simulink library "component_lib"  (R2023a)
settings: Solver=VariableStepAuto  StartTime=0.0  StopTime=10.0  RelTol=1e-3
undefined symbols (not defined in the file or in its folder): ECCV_r, par, R1234yf_ph, V_nom
libraries: base_lib x258, $bdroot x212, simulink x2, slpidlib x1
(part 6 of 7)

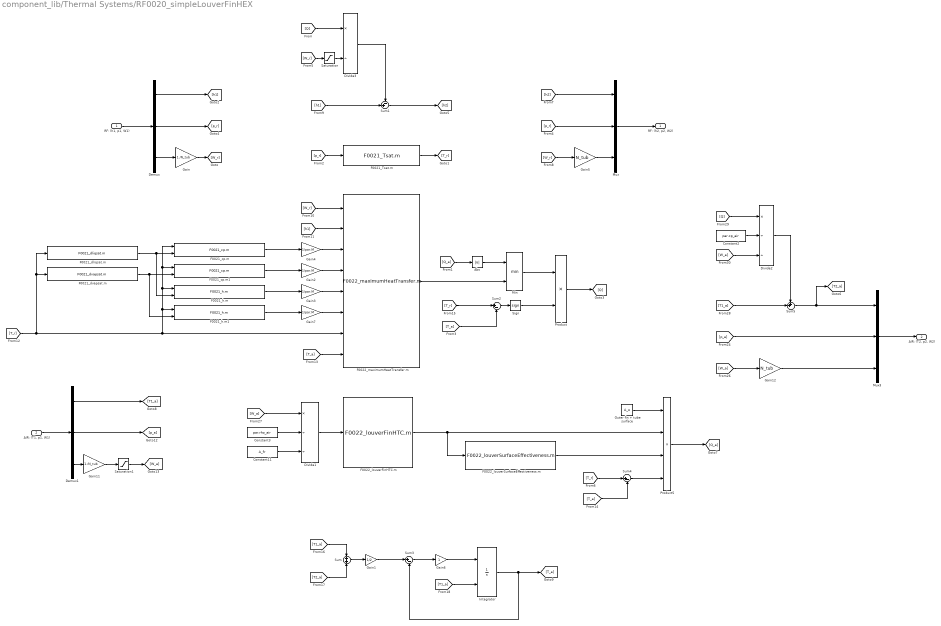
== system component_lib/Thermal Systems/RF0020_simpleLouverFinHEX ==
  "RF: (h1, p1, W1)" : Inport
  "AIR: (T1, p1, W1)" : Inport  Port=2
  Abs : Abs  SaturateOnIntegerOverflow=off
  Constant11 : Constant  Value=A_fr
  Constant2 : Constant  Value=par.cp_air
  Constant3 : Constant  Value=par.rho_air
  Demux : Demux  Outputs=3
  Demux1 : Demux  Outputs=3
  Divide1 : Product  Inputs=*//
  Divide2 : Product  Inputs=*//
  Divide3 : Product  Inputs=*/
  F0021_Tsat.m : base_lib/F0021_R1234yf/F0021_Tsat.m  SystemSampleTime=-1  VariantActivationTime=update diagram  Latency=0  AutoFrameSizeCalculation=off
      settings: LibrarySourceBlock=|
      | simulink/User-Defined
      | Functions/MATLAB Function
  F0021_cp.m : base_lib/F0021_R1234yf/F0021_cp.m  SystemSampleTime=-1  VariantActivationTime=update diagram  Latency=0  AutoFrameSizeCalculation=off
      settings: LibrarySourceBlock=|
      | simulink/User-Defined
      | Functions/MATLAB Function
  F0021_cp.m1 : base_lib/F0021_R1234yf/F0021_cp.m  SystemSampleTime=-1  VariantActivationTime=update diagram  Latency=0  AutoFrameSizeCalculation=off
      settings: LibrarySourceBlock=|
      | simulink/User-Defined
      | Functions/MATLAB Function
  F0021_dliqsat.m : base_lib/F0021_R1234yf/F0021_dliqsat.m  SystemSampleTime=-1  VariantActivationTime=update diagram  Latency=0  AutoFrameSizeCalculation=off
      settings: LibrarySourceBlock=|
      | simulink/User-Defined
      | Functions/MATLAB Function
  F0021_dvapsat.m : base_lib/F0021_R1234yf/F0021_dvapsat.m  SystemSampleTime=-1  VariantActivationTime=update diagram  Latency=0  AutoFrameSizeCalculation=off
      settings: LibrarySourceBlock=|
      | simulink/User-Defined
      | Functions/MATLAB Function
  F0021_h.m : base_lib/F0021_R1234yf/F0021_h.m  SystemSampleTime=-1  VariantActivationTime=update diagram  Latency=0  AutoFrameSizeCalculation=off
      settings: LibrarySourceBlock=|
      | simulink/User-Defined
      | Functions/MATLAB Function
  F0021_h.m1 : base_lib/F0021_R1234yf/F0021_h.m  SystemSampleTime=-1  VariantActivationTime=update diagram  Latency=0  AutoFrameSizeCalculation=off
      settings: LibrarySourceBlock=|
      | simulink/User-Defined
      | Functions/MATLAB Function
  F0022_louverFinHTC.m : base_lib/F0022_heatPump/F0022_louverFinHTC.m  SystemSampleTime=-1  VariantActivationTime=update diagram  Latency=0  AutoFrameSizeCalculation=off
      settings: LibrarySourceBlock=|
      | simulink/User-Defined
      | Functions/MATLAB Function
  F0022_louverSurfaceEffectiveness.m : base_lib/F0022_heatPump/F0022_louverSurfaceEffectiveness.m  SystemSampleTime=-1  VariantActivationTime=update diagram  Latency=0  AutoFrameSizeCalculation=off
      settings: LibrarySourceBlock=|
      | simulink/User-Defined
      | Functions/MATLAB Function
  F0022_maximumHeatTransfer.m : base_lib/F0022_heatPump/F0022_maximumHeatTransfer.m  SystemSampleTime=-1  VariantActivationTime=update diagram  Latency=0  AutoFrameSizeCalculation=off
      settings: LibrarySourceBlock=|
      | simulink/User-Defined
      | Functions/MATLAB Function
  Gain : Gain  Gain=1./N_tub
  Gain1 : Gain  Gain=1/2
  Gain11 : Gain  Gain=1./N_tub
  Gain12 : Gain  Gain=N_tub
  Gain{2..4,7} (4 alike) : Gain  Gain=1/par.M
  Gain5 : Gain  Gain=N_tub
  Gain6 : Gain
  Integrator : Integrator  InitialConditionSource=external  LimitOutput=on  UpperSaturationLimit=273+100  LowerSaturationLimit=273-40
  Min : MinMax  Inputs=2
  Mux : Mux  Inputs=3
  Mux3 : Mux  Inputs=3
  Outer fin + tube surface : Constant  Value=A_o
  Product : Product
  Product5 : Product  Inputs=4
  Saturation : Saturate  UpperLimit=inf  LowerLimit=1e-5
  Saturation1 : Saturate  UpperLimit=inf  LowerLimit=1e-3
  Sign : Signum
  Sum : Sum  Inputs=+|+
  Sum1 : Sum  Inputs=-+|
  Sum2 : Sum  Inputs=|+-
  Sum3 : Sum  Inputs=|+-
  Sum4 : Sum  Inputs=|+-
  Sum5 : Sum  Inputs=++|
  "RF: (h2, p2, W2)" : Outport
  "AIR: (T2, p2, W2)" : Outport  Port=2
  wires:
  [h2] -> Mux/1
  Gain5/1 -> Mux/3
  Demux/1 -> [h1]
  Demux/3 -> Gain/1
  Mux3/1 -> "AIR: (T2, p2, W2)"/1
  "AIR: (T1, p1, W1)"/1 -> Demux1/1
  Gain/1 -> [W_r]
  [p_r] -> Mux/2
  Demux/2 -> [p_r]
  [W_r] -> Gain5/1
  Mux/1 -> "RF: (h2, p2, W2)"/1
  "RF: (h1, p1, W1)"/1 -> Demux/1
  F0022_louverFinHTC.m/1 -> Product5/2, F0022_louverSurfaceEffectiveness.m/1
  Divide1/1 -> F0022_louverFinHTC.m/1
  Constant3/1 -> Divide1/2
  Constant11/1 -> Divide1/3
  Product5/1 -> [Q_a]
  Outer fin + tube surface/1 -> Product5/1
  [T_a] -> Sum4/2
  Sum4/1 -> Product5/4
  F0022_louverSurfaceEffectiveness.m/1 -> Product5/3
  Demux1/1 -> [T1_a]
  Demux1/2 -> [p_a]
  [p_a] -> Mux3/2
  Demux1/3 -> Gain11/1
  [W_a] -> Divide1/1
  Gain12/1 -> Mux3/3
  Gain11/1 -> Saturation1/1
  [W_a] -> Gain12/1
  [T1_a] -> Sum5/2
  Sum5/1 -> [T2_a], Mux3/1
  [Q] -> Divide2/1
  Constant2/1 -> Divide2/2
  [W_a] -> Divide2/3
  Divide2/1 -> Sum5/1
  Saturation1/1 -> [W_a]
  [p_r] -> F0021_Tsat.m/1
  F0021_Tsat.m/1 -> [T_r]
  [T_r] -> Sum4/1
  [Q] -> Divide3/1
  [h1] -> Sum1/2
  Divide3/1 -> Sum1/1
  Sum1/1 -> [h2]
  [W_r] -> F0022_maximumHeatTransfer.m/1
  [h1] -> F0022_maximumHeatTransfer.m/2
  Gain4/1 -> F0022_maximumHeatTransfer.m/3
  Gain2/1 -> F0022_maximumHeatTransfer.m/4
  F0021_cp.m/1 -> Gain4/1
  F0021_cp.m1/1 -> Gain2/1
  F0021_dliqsat.m/1 -> F0021_h.m/2, F0021_cp.m/2
  F0021_dvapsat.m/1 -> F0021_h.m1/2, F0021_cp.m1/2
  [T_r] -> F0021_dliqsat.m/1, F0021_dvapsat.m/1, F0021_cp.m/1, F0021_cp.m1/1, F0021_h.m/1, F0021_h.m1/1, F0022_maximumHeatTransfer.m/7
  Gain3/1 -> F0022_maximumHeatTransfer.m/5
  F0021_h.m/1 -> Gain3/1
  F0021_h.m1/1 -> Gain7/1
  Gain7/1 -> F0022_maximumHeatTransfer.m/6
  [T_a] -> F0022_maximumHeatTransfer.m/8
  F0022_maximumHeatTransfer.m/1 -> Min/2
  [Q_a] -> Abs/1
  Abs/1 -> Min/1
  [T_a] -> Sum2/2
  [T_r] -> Sum2/1
  Sum2/1 -> Sign/1
  Min/1 -> Product/1
  Sign/1 -> Product/2
  Product/1 -> [Q]
  [T2_a] -> Sum/2
  [T1_a] -> Sum/1
  Sum/1 -> Gain1/1
  Gain1/1 -> Sum3/1
  Sum3/1 -> Gain6/1
  Gain6/1 -> Integrator/1
  Integrator/1 -> [T_a], Sum3/2
  [T1_a] -> Integrator/2
  [W_r] -> Saturation/1
  Saturation/1 -> Divide3/2

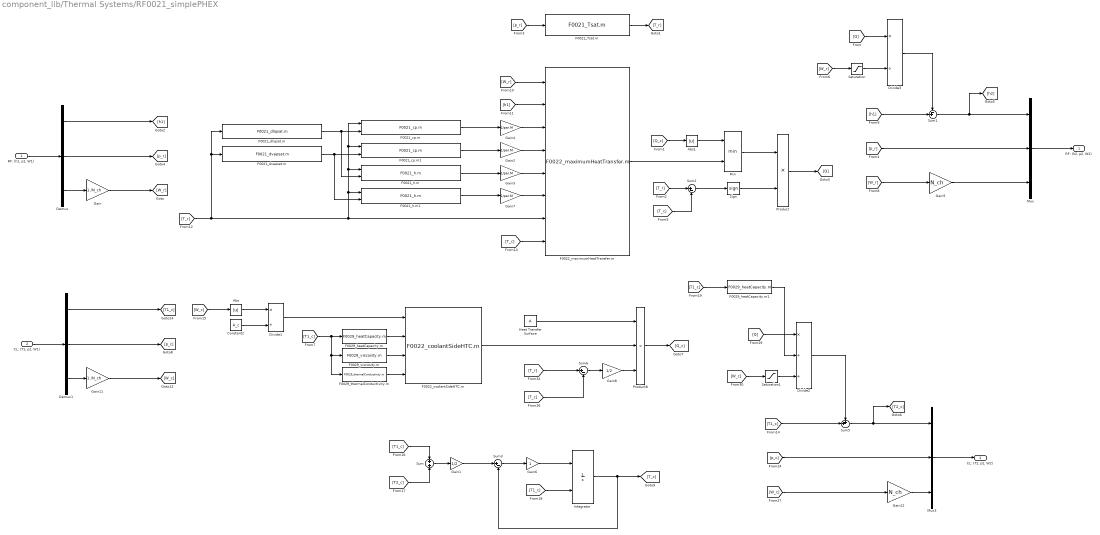
== system component_lib/Thermal Systems/RF0021_simplePHEX ==
  "RF: (h1, p1, W1)" : Inport
  "CL: (T1, p1, W1)" : Inport  Port=2
  Abs : Abs  SaturateOnIntegerOverflow=off
  Abs1 : Abs  SaturateOnIntegerOverflow=off
  Constant2 : Constant  Value=A_c
  Demux : Demux  Outputs=3
  Demux1 : Demux  Outputs=3
  Divide1 : Product  Inputs=*/
  Divide2 : Product  Inputs=*//
  Divide3 : Product  Inputs=*/
  F0021_Tsat.m : base_lib/F0021_R1234yf/F0021_Tsat.m  SystemSampleTime=-1  VariantActivationTime=update diagram  Latency=0  AutoFrameSizeCalculation=off
      settings: LibrarySourceBlock=|
      | simulink/User-Defined
      | Functions/MATLAB Function
  F0021_cp.m : base_lib/F0021_R1234yf/F0021_cp.m  SystemSampleTime=-1  VariantActivationTime=update diagram  Latency=0  AutoFrameSizeCalculation=off
      settings: LibrarySourceBlock=|
      | simulink/User-Defined
      | Functions/MATLAB Function
  F0021_cp.m1 : base_lib/F0021_R1234yf/F0021_cp.m  SystemSampleTime=-1  VariantActivationTime=update diagram  Latency=0  AutoFrameSizeCalculation=off
      settings: LibrarySourceBlock=|
      | simulink/User-Defined
      | Functions/MATLAB Function
  F0021_dliqsat.m : base_lib/F0021_R1234yf/F0021_dliqsat.m  SystemSampleTime=-1  VariantActivationTime=update diagram  Latency=0  AutoFrameSizeCalculation=off
      settings: LibrarySourceBlock=|
      | simulink/User-Defined
      | Functions/MATLAB Function
  F0021_dvapsat.m : base_lib/F0021_R1234yf/F0021_dvapsat.m  SystemSampleTime=-1  VariantActivationTime=update diagram  Latency=0  AutoFrameSizeCalculation=off
      settings: LibrarySourceBlock=|
      | simulink/User-Defined
      | Functions/MATLAB Function
  F0021_h.m : base_lib/F0021_R1234yf/F0021_h.m  SystemSampleTime=-1  VariantActivationTime=update diagram  Latency=0  AutoFrameSizeCalculation=off
      settings: LibrarySourceBlock=|
      | simulink/User-Defined
      | Functions/MATLAB Function
  F0021_h.m1 : base_lib/F0021_R1234yf/F0021_h.m  SystemSampleTime=-1  VariantActivationTime=update diagram  Latency=0  AutoFrameSizeCalculation=off
      settings: LibrarySourceBlock=|
      | simulink/User-Defined
      | Functions/MATLAB Function
  F0022_coolantSideHTC.m : base_lib/F0022_heatPump/F0022_coolantSideHTC.m  SystemSampleTime=-1  VariantActivationTime=update diagram  Latency=0  AutoFrameSizeCalculation=off
      settings: LibrarySourceBlock=|
      | simulink/User-Defined
      | Functions/MATLAB Function
  F0022_maximumHeatTransfer.m : base_lib/F0022_heatPump/F0022_maximumHeatTransfer.m  SystemSampleTime=-1  VariantActivationTime=update diagram  Latency=0  AutoFrameSizeCalculation=off
      settings: LibrarySourceBlock=|
      | simulink/User-Defined
      | Functions/MATLAB Function
  F0029_heatCapacity.m : base_lib/F0029_coolantWrapper/F0029_heatCapacity.m  SystemSampleTime=-1  VariantActivationTime=update diagram  Latency=0  AutoFrameSizeCalculation=off
      settings: LibrarySourceBlock=|
      | simulink/User-Defined
      | Functions/MATLAB Function
  F0029_heatCapacity.m1 : base_lib/F0029_coolantWrapper/F0029_heatCapacity.m  SystemSampleTime=-1  VariantActivationTime=update diagram  Latency=0  AutoFrameSizeCalculation=off
      settings: LibrarySourceBlock=|
      | simulink/User-Defined
      | Functions/MATLAB Function
  F0029_thermalConductivity.m : base_lib/F0029_coolantWrapper/F0029_thermalConductivity.m  SystemSampleTime=-1  VariantActivationTime=update diagram  Latency=0  AutoFrameSizeCalculation=off
      settings: LibrarySourceBlock=|
      | simulink/User-Defined
      | Functions/MATLAB Function
  F0029_viscosity.m : base_lib/F0029_coolantWrapper/F0029_viscosity.m  SystemSampleTime=-1  VariantActivationTime=update diagram  Latency=0  AutoFrameSizeCalculation=off
      settings: LibrarySourceBlock=|
      | simulink/User-Defined
      | Functions/MATLAB Function
  Gain : Gain  Gain=1./N_ch
  Gain1 : Gain  Gain=1/2
  Gain11 : Gain  Gain=1./N_ch
  Gain12 : Gain  Gain=N_ch
  Gain{2..4,7} (4 alike) : Gain  Gain=1/par.M
  Gain5 : Gain  Gain=N_ch
  Gain6 : Gain
  Gain8 : Gain  Gain=1/2
  Heat Transfer Surface : Constant  Value=A
  Integrator : Integrator  InitialConditionSource=external  LimitOutput=on  UpperSaturationLimit=273+100  LowerSaturationLimit=273-40
  Min : MinMax  Inputs=2
  Mux : Mux  Inputs=3
  Mux3 : Mux  Inputs=3
  Product : Product
  Product8 : Product  Inputs=3
  Saturation : Saturate  UpperLimit=inf  LowerLimit=0.0001
  Saturation1 : Saturate  UpperLimit=inf  LowerLimit=0.0001
  Sign : Signum
  Sum : Sum  Inputs=+|+
  Sum1 : Sum  Inputs=-+|
  Sum2 : Sum  Inputs=|+-
  Sum3 : Sum  Inputs=|+-
  Sum5 : Sum  Inputs=++|
  Sum6 : Sum  Inputs=|+-
  "RF: (h2, p2, W2)" : Outport
  "CL: (T2, p2, W2)" : Outport  Port=2
  wires:
  "RF: (h1, p1, W1)"/1 -> Demux/1
  Mux/1 -> "RF: (h2, p2, W2)"/1
  [W_r] -> Gain5/1
  [p_r] -> Mux/2
  Gain/1 -> [W_r]
  "CL: (T1, p1, W1)"/1 -> Demux1/1
  [p_c] -> Mux3/2
  Mux3/1 -> "CL: (T2, p2, W2)"/1
  Divide1/1 -> F0022_coolantSideHTC.m/1
  Product8/1 -> [Q_c]
  Sum6/1 -> Gain8/1
  [T_c] -> Sum6/2
  Demux1/2 -> [p_c]
  [T_r] -> Sum6/1
  Heat Transfer Surface/1 -> Product8/1
  Demux/3 -> Gain/1
  Demux/1 -> [h1]
  Gain5/1 -> Mux/3
  Sum1/1 -> Mux/1, [h2]
  Gain12/1 -> Mux3/3
  Demux1/3 -> Gain11/1
  Demux1/1 -> [T1_c]
  Abs/1 -> Divide1/1
  Constant2/1 -> Divide1/2
  [W_c] -> Abs/1
  Demux/2 -> [p_r]
  Sign/1 -> Product/2
  F0021_cp.m1/1 -> Gain2/1
  Gain2/1 -> F0022_maximumHeatTransfer.m/4
  [T_c] -> Sum2/2
  [T_r] -> Sum2/1
  F0021_h.m1/1 -> Gain7/1
  [T_r] -> F0021_dliqsat.m/1, F0021_dvapsat.m/1, F0021_cp.m/1, F0021_cp.m1/1, F0021_h.m/1, F0021_h.m1/1, F0022_maximumHeatTransfer.m/7
  [W_r] -> F0022_maximumHeatTransfer.m/1
  [W_r] -> Saturation/1
  [Q] -> Divide3/1
  Gain4/1 -> F0022_maximumHeatTransfer.m/3
  [p_r] -> F0021_Tsat.m/1
  Gain3/1 -> F0022_maximumHeatTransfer.m/5
  F0021_dvapsat.m/1 -> F0021_h.m1/2, F0021_cp.m1/2
  Product/1 -> [Q]
  [Q_c] -> Abs1/1
  F0022_maximumHeatTransfer.m/1 -> Min/2
  Min/1 -> Product/1
  F0021_h.m/1 -> Gain3/1
  Gain7/1 -> F0022_maximumHeatTransfer.m/6
  Abs1/1 -> Min/1
  Divide3/1 -> Sum1/1
  F0021_Tsat.m/1 -> [T_r]
  F0021_cp.m/1 -> Gain4/1
  F0021_dliqsat.m/1 -> F0021_h.m/2, F0021_cp.m/2
  [h1] -> F0022_maximumHeatTransfer.m/2
  Sum2/1 -> Sign/1
  [T_c] -> F0022_maximumHeatTransfer.m/8
  Gain6/1 -> Integrator/1
  Sum/1 -> Gain1/1
  Gain1/1 -> Sum3/1
  Integrator/1 -> [T_c], Sum3/2
  Sum3/1 -> Gain6/1
  [T2_c] -> Sum/2
  [T1_c] -> Sum/1
  [T1_c] -> Integrator/2
  [Q] -> Divide2/1
  F0029_heatCapacity.m1/1 -> Divide2/2
  Divide2/1 -> Sum5/1
  [T1_c] -> Sum5/2
  Sum5/1 -> Mux3/1, [T2_c]
  [h1] -> Sum1/2
  F0022_coolantSideHTC.m/1 -> Product8/2
  Gain11/1 -> [W_c]
  [W_c] -> Gain12/1
  Gain8/1 -> Product8/3
  Saturation/1 -> Divide3/2
  [W_c] -> Saturation1/1
  Saturation1/1 -> Divide2/3
  [T1_c] -> F0029_thermalConductivity.m/1, F0029_viscosity.m/1, F0029_heatCapacity.m/1
  F0029_heatCapacity.m/1 -> F0022_coolantSideHTC.m/2
  F0029_viscosity.m/1 -> F0022_coolantSideHTC.m/3
  F0029_thermalConductivity.m/1 -> F0022_coolantSideHTC.m/4
  [T1_c] -> F0029_heatCapacity.m1/1

== system component_lib/Thermal Systems/RF0022_simpleExpansionValve ==
  exv [-] : Inport
  "RF: (h1, p1, W)" : Inport  Port=2
  Demux : Demux  Outputs=3
  Density Look-up : Lookup_n-D  BreakpointsForDimension1=R1234yf_ph.p  BreakpointsForDimension2=R1234yf_ph.h  Table=R1234yf_ph.D  InternalRulePriority=Speed  RndMeth=Simplest
      settings: InputPortMap=u0,u1
  F0022_simpleExpansionValve.m : base_lib/F0022_heatPump/F0022_simpleExpansionValve.m  SystemSampleTime=-1  VariantActivationTime=update diagram  Latency=0  AutoFrameSizeCalculation=off
      settings: LibrarySourceBlock=|
      | simulink/User-Defined
      | Functions/MATLAB Function
  Gain1 : Gain  Gain=par.M
  Gain6 : Gain  Gain=par.M
  Mux : Mux  Inputs=3
  Saturation : Saturate  UpperLimit=1  LowerLimit=0
  Saturation3 : Saturate  UpperLimit=inf  LowerLimit=p_min
  Sum : Sum  Inputs=|+-
  Transfer Fcn : TransferFcn  Denominator=[1 1]
  dp [Pa] : Outport
  "RF: (h2, p2, W2)" : Outport  Port=2
  wires:
  Gain1/1 -> Density Look-up/2
  Density Look-up/1 -> Gain6/1
  [h_1] -> Gain1/1
  exv [-]/1 -> Saturation/1
  Gain6/1 -> F0022_simpleExpansionValve.m/2
  Saturation/1 -> F0022_simpleExpansionValve.m/3
  [p_1] -> Density Look-up/1
  F0022_simpleExpansionValve.m/1 -> dp [Pa]/1, Transfer Fcn/1
  "RF: (h1, p1, W)"/1 -> Demux/1
  Demux/2 -> [p_1]
  Demux/3 -> [W]
  Demux/1 -> [h2], [h_1]
  [W] -> F0022_simpleExpansionValve.m/1
  Mux/1 -> "RF: (h2, p2, W2)"/1
  [W] -> Mux/3
  [h2] -> Mux/1
  Transfer Fcn/1 -> Sum/2
  [p_1] -> Sum/1
  Sum/1 -> Saturation3/1
  Saturation3/1 -> Mux/2

== system component_lib/Thermal Systems/RF0022_valve ==
  open [-] : Inport
  A: (h1,p1,W1) : Inport  Port=2
  split [-] : Inport  Port=3
  Constant : Constant  Value=par.d
  Constant1 : Constant
  Constant2 : Constant
  Constant3 : Constant  Value=par.d
  Demux : Demux  Outputs=3
  Density Look-up : Lookup_n-D  BreakpointsForDimension1=R1234yf_ph.p  BreakpointsForDimension2=R1234yf_ph.h  Table=R1234yf_ph.D  InternalRulePriority=Speed  RndMeth=Simplest
      settings: InputPortMap=u0,u1
  F0022_incompressibleRestriction.m : base_lib/F0022_heatPump/F0022_incompressibleRestriction.m  SystemSampleTime=-1  VariantActivationTime=update diagram  Latency=0  AutoFrameSizeCalculation=off
      settings: LibrarySourceBlock=|
      | simulink/User-Defined
      | Functions/MATLAB Function
  F0022_incompressibleRestriction.m1 : base_lib/F0022_heatPump/F0022_incompressibleRestriction.m  SystemSampleTime=-1  VariantActivationTime=update diagram  Latency=0  AutoFrameSizeCalculation=off
      settings: LibrarySourceBlock=|
      | simulink/User-Defined
      | Functions/MATLAB Function
  Gain3 : Gain  Gain=par.M
  Gain5 : Gain  Gain=par.M
  Mux : Mux  Inputs=3
  Mux1 : Mux  Inputs=3
  Product{,1..3} (4 alike) : Product
  Saturation : Saturate  UpperLimit=1  LowerLimit=0
  Saturation1 : Saturate  UpperLimit=0.99  LowerLimit=0.01
  Sum : Sum  Inputs=-+|
  Sum1 : Sum  Inputs=-+|
  Sum2 : Sum  Inputs=|+-
  Sum3 : Sum  Inputs=|+-
  Transfer Fcn : TransferFcn  Denominator=[0.1 1]
  B: (h2,p2,W2) : Outport
  C: (h3,p3,W3) : Outport  Port=2
  wires:
  A: (h1,p1,W1)/1 -> Demux/1
  Mux/1 -> B: (h2,p2,W2)/1
  Saturation1/1 -> Sum/1, Product/1
  Constant1/1 -> Sum/2
  Sum/1 -> Product1/2
  Constant2/1 -> Sum1/2
  Product2/1 -> [W_21], F0022_incompressibleRestriction.m/1
  Product3/1 -> F0022_incompressibleRestriction.m1/1, [W_20]
  Sum1/1 -> Product3/2
  Demux/3 -> Product3/1, Product2/1
  Mux1/1 -> C: (h3,p3,W3)/1
  Sum2/1 -> Mux/2
  F0022_incompressibleRestriction.m/1 -> Sum2/2
  [W_20] -> Mux1/3
  Demux/2 -> [p_1]
  Sum3/1 -> Mux1/2
  [p_1] -> Sum3/1
  F0022_incompressibleRestriction.m1/1 -> Sum3/2
  [p_1] -> Sum2/1
  [W_21] -> Mux/3
  Saturation/1 -> Sum1/1, Product2/2
  split [-]/1 -> Saturation/1
  open [-]/1 -> Transfer Fcn/1
  Transfer Fcn/1 -> Saturation1/1
  Constant/1 -> Product/2
  Constant3/1 -> Product1/1
  Product/1 -> F0022_incompressibleRestriction.m/2
  Product1/1 -> F0022_incompressibleRestriction.m1/2
  Density Look-up/1 -> Gain5/1
  [p_1] -> Density Look-up/1
  Gain5/1 -> [rho]
  Gain3/1 -> Density Look-up/2
  Demux/1 -> Mux1/1, Mux/1, Gain3/1
  [rho] -> F0022_incompressibleRestriction.m/3
  [rho] -> F0022_incompressibleRestriction.m1/3

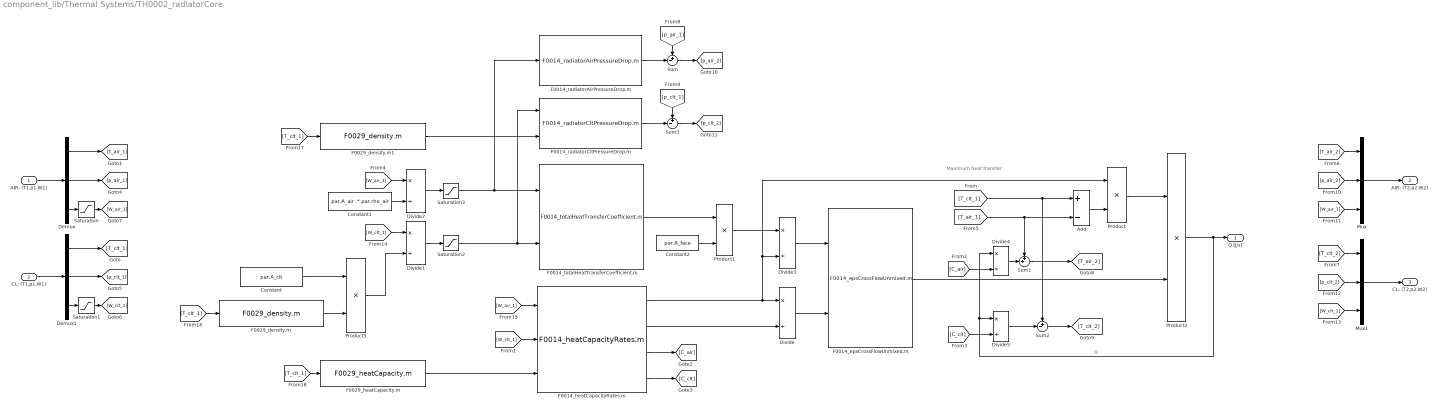
== system component_lib/Thermal Systems/TH0002_radiatorCore ==
  note: Maximum heat transfer
  AIR: (T1,p1,W1) : Inport
  CL: (T1,p1,W1) : Inport  Port=2
  Add : Sum  Inputs=+-
  Constant : Constant  Value=par.A_clt
  Constant1 : Constant  Value=par.A_air .* par.rho_air
  Constant2 : Constant  Value=par.A_face
  Demux : Demux  Outputs=3
  Demux1 : Demux  Outputs=3
  Divide{,1..5} (6 alike) : Product  Inputs=*/
  F0014_epsCrossFlowUnmixed.m : base_lib/F0014_titanXradiator/F0014_epsCrossFlowUnmixed.m  SystemSampleTime=-1  VariantActivationTime=update diagram  Latency=0  AutoFrameSizeCalculation=off
      settings: LibrarySourceBlock=|
      | simulink/User-Defined
      | Functions/MATLAB Function
  F0014_heatCapacityRates.m : base_lib/F0014_titanXradiator/F0014_heatCapacityRates.m  SystemSampleTime=-1  VariantActivationTime=update diagram  Latency=0  AutoFrameSizeCalculation=off
      settings: LibrarySourceBlock=|
      | simulink/User-Defined
      | Functions/MATLAB Function
  F0014_radiatorAirPressureDrop.m : base_lib/F0014_titanXradiator/F0014_radiatorAirPressureDrop.m  SystemSampleTime=-1  VariantActivationTime=update diagram  Latency=0  AutoFrameSizeCalculation=off
      settings: LibrarySourceBlock=|
      | simulink/User-Defined
      | Functions/MATLAB Function
  F0014_radiatorCltPressureDrop.m : base_lib/F0014_titanXradiator/F0014_radiatorCltPressureDrop.m  SystemSampleTime=-1  VariantActivationTime=update diagram  Latency=0  AutoFrameSizeCalculation=off
      settings: LibrarySourceBlock=|
      | simulink/User-Defined
      | Functions/MATLAB Function
  F0014_totalHeatTransferCoefficient.m : base_lib/F0014_titanXradiator/F0014_totalHeatTransferCoefficient.m  SystemSampleTime=-1  VariantActivationTime=update diagram  Latency=0  AutoFrameSizeCalculation=off
      settings: LibrarySourceBlock=|
      | simulink/User-Defined
      | Functions/MATLAB Function
  F0029_density.m : base_lib/F0029_coolantWrapper/F0029_density.m  SystemSampleTime=-1  VariantActivationTime=update diagram  Latency=0  AutoFrameSizeCalculation=off
      settings: LibrarySourceBlock=|
      | simulink/User-Defined
      | Functions/MATLAB Function
  F0029_density.m1 : base_lib/F0029_coolantWrapper/F0029_density.m  SystemSampleTime=-1  VariantActivationTime=update diagram  Latency=0  AutoFrameSizeCalculation=off
      settings: LibrarySourceBlock=|
      | simulink/User-Defined
      | Functions/MATLAB Function
  F0029_heatCapacity.m : base_lib/F0029_coolantWrapper/F0029_heatCapacity.m  SystemSampleTime=-1  VariantActivationTime=update diagram  Latency=0  AutoFrameSizeCalculation=off
      settings: LibrarySourceBlock=|
      | simulink/User-Defined
      | Functions/MATLAB Function
  Mux : Mux  Inputs=3
  Mux1 : Mux  Inputs=3
  Product{,1..3} (4 alike) : Product
  Saturation : Saturate  UpperLimit=inf  LowerLimit=1e-5
  Saturation1 : Saturate  UpperLimit=inf  LowerLimit=1e-5
  Saturation2 : Saturate  UpperLimit=inf  LowerLimit=1e-3
  Saturation3 : Saturate  UpperLimit=inf  LowerLimit=1e-3
  Sum : Sum  Inputs=+-|
  Sum1 : Sum  Inputs=++|
  Sum2 : Sum  Inputs=+-|
  Sum3 : Sum  Inputs=+-|
  Q [J/s] : Outport
  AIR: (T2,p2,W2) : Outport  Port=2
  CL: (T2,p2,W2) : Outport  Port=3
  wires:
  F0014_heatCapacityRates.m/2 -> Divide/2
  F0014_heatCapacityRates.m/1 -> Product/1, Divide3/2, Divide/1
  Divide/1 -> F0014_epsCrossFlowUnmixed.m/2
  Constant/1 -> Product3/1
  Divide1/1 -> Saturation2/1
  [W_air_1] -> Divide2/1
  Constant1/1 -> Divide2/2
  Divide2/1 -> Saturation3/1
  F0014_totalHeatTransferCoefficient.m/1 -> Product1/1
  Constant2/1 -> Product1/2
  Product1/1 -> Divide3/1
  Divide3/1 -> F0014_epsCrossFlowUnmixed.m/1
  F0014_epsCrossFlowUnmixed.m/1 -> Product2/2
  Add/1 -> Product/2
  Product2/1 -> Q [J/s]/1, Divide4/1, Divide5/1  "Q"
  [T_clt_1] -> Sum2/1, Add/1
  Product/1 -> Product2/1
  F0014_heatCapacityRates.m/3 -> [C_air]
  F0014_heatCapacityRates.m/4 -> [C_clt]
  [T_air_1] -> Add/2, Sum1/1
  Divide4/1 -> Sum1/2
  [C_air] -> Divide4/2
  [C_clt] -> Divide5/2
  Divide5/1 -> Sum2/2
  AIR: (T1,p1,W1)/1 -> Demux/1
  CL: (T1,p1,W1)/1 -> Demux1/1
  Demux1/1 -> [T_clt_1]
  Demux/1 -> [T_air_1]
  Demux/2 -> [p_air_1]
  Demux1/2 -> [p_clt_1]
  Sum1/1 -> [T_air_2]
  Sum2/1 -> [T_clt_2]
  Mux/1 -> AIR: (T2,p2,W2)/1
  [p_air_1] -> Sum/1
  F0014_radiatorAirPressureDrop.m/1 -> Sum/2
  Sum/1 -> [p_air_2]
  Sum3/1 -> [p_clt_2]
  F0014_radiatorCltPressureDrop.m/1 -> Sum3/2
  [p_clt_1] -> Sum3/1
  [T_clt_2] -> Mux1/1
  [T_air_2] -> Mux/1
  [p_air_2] -> Mux/2
  [W_air_1] -> Mux/3
  [p_clt_2] -> Mux1/2
  [W_clt_1] -> Mux1/3
  Mux1/1 -> CL: (T2,p2,W2)/1
  Demux1/3 -> Saturation1/1
  Saturation1/1 -> [W_clt_1]
  Demux/3 -> Saturation/1
  Saturation/1 -> [W_air_1]
  [W_clt_1] -> F0014_heatCapacityRates.m/2
  [W_clt_1] -> Divide1/1
  [W_air_1] -> F0014_heatCapacityRates.m/1
  Saturation2/1 -> F0014_radiatorCltPressureDrop.m/1, F0014_totalHeatTransferCoefficient.m/2
  Saturation3/1 -> F0014_radiatorAirPressureDrop.m/1, F0014_totalHeatTransferCoefficient.m/1
  F0029_density.m/1 -> Product3/2
  Product3/1 -> Divide1/2
  [T_clt_1] -> F0029_density.m/1
  [T_clt_1] -> F0029_density.m1/1
  F0029_density.m1/1 -> F0014_radiatorCltPressureDrop.m/2
  F0029_heatCapacity.m/1 -> F0014_heatCapacityRates.m/3
  [T_clt_1] -> F0029_heatCapacity.m/1

== system component_lib/Thermal Systems/TH0003_coolantTank ==
  CL: (T1,p1,W1) : Inport
  Demux1 : Demux  Outputs=3
  Divide : Product  Inputs=*/
  F0014_tankPressureDrop.m : base_lib/F0014_titanXradiator/F0014_tankPressureDrop.m  SystemSampleTime=-1  VariantActivationTime=update diagram  Latency=0  AutoFrameSizeCalculation=off
      settings: LibrarySourceBlock=|
      | simulink/User-Defined
      | Functions/MATLAB Function
  F0029_density.m : base_lib/F0029_coolantWrapper/F0029_density.m  SystemSampleTime=-1  VariantActivationTime=update diagram  Latency=0  AutoFrameSizeCalculation=off
      settings: LibrarySourceBlock=|
      | simulink/User-Defined
      | Functions/MATLAB Function
  Integrator : Integrator  InitialCondition=T_0
  Mixing/Mass factor - empirical : Gain  Gain=3
  Mux1 : Mux  Inputs=3
  Product : Product
  Product1 : Product
  Product3 : Product  Inputs=*/
  Product5 : Product  Inputs=*/
  Subtract : Sum  Inputs=+-
  Sum : Sum  Inputs=|+-
  Tank volume : Constant  Value=par.V
  connector inlet area : Constant  Value=par.A_con
  CL: (T2,p2,W2) : Outport
  wires:
  CL: (T1,p1,W1)/1 -> Demux1/1
  Demux1/3 -> [W_clt_1]
  Demux1/1 -> [T_clt_1]
  Demux1/2 -> [p_clt_1]
  Mux1/1 -> CL: (T2,p2,W2)/1
  [p_clt_2] -> Mux1/2
  [W_clt_1] -> Mux1/3
  [T_clt_2] -> Mux1/1
  Tank volume/1 -> Mixing/Mass factor - empirical/1
  [W_clt_1] -> Product5/1
  [p_clt_1] -> Sum/1
  [T_clt_1] -> Subtract/1
  [W_clt_1] -> Product1/2
  Subtract/1 -> Product1/1
  Integrator/1 -> [T_clt_2], Subtract/2
  Mixing/Mass factor - empirical/1 -> Product/1
  Product/1 -> Divide/2
  Product1/1 -> Divide/1
  connector inlet area/1 -> Product3/2
  Sum/1 -> [p_clt_2]
  Product5/1 -> Product3/1
  Divide/1 -> Integrator/1
  F0014_tankPressureDrop.m/1 -> Sum/2
  Product3/1 -> F0014_tankPressureDrop.m/1  "v"
  F0029_density.m/1 -> Product/2, Product5/2
  [T_clt_1] -> F0029_density.m/1

== system component_lib/Thermal Systems/TH0004_radiatorPlugFlow ==
  CL: (T1,p1,W1) : Inport
  Demux1 : Demux  Outputs=3
  F0014_coreFlowDelay.m : base_lib/F0014_titanXradiator/F0014_coreFlowDelay.m  SystemSampleTime=-1  VariantActivationTime=update diagram  Latency=0  AutoFrameSizeCalculation=off
      settings: LibrarySourceBlock=|
      | simulink/User-Defined
      | Functions/MATLAB Function
  F0029_density.m : base_lib/F0029_coolantWrapper/F0029_density.m  SystemSampleTime=-1  VariantActivationTime=update diagram  Latency=0  AutoFrameSizeCalculation=off
      settings: LibrarySourceBlock=|
      | simulink/User-Defined
      | Functions/MATLAB Function
  Mux1 : Mux  Inputs=3
  Saturation1 : Saturate  UpperLimit=inf  LowerLimit=1e-5
  Variable Transport Delay1 : VariableTransportDelay  VariableDelayType=Variable transport delay  MaximumDelay=20  InitialOutput=T_0  MaximumPoints=10240  TransDelayFeedthrough=on
  CL: (T2,p2,W2) : Outport
  wires:
  F0014_coreFlowDelay.m/1 -> Variable Transport Delay1/2
  Variable Transport Delay1/1 -> Mux1/1
  CL: (T1,p1,W1)/1 -> Demux1/1
  Demux1/3 -> Saturation1/1
  Demux1/2 -> [p_clt_1]
  Demux1/1 -> F0029_density.m/1, Variable Transport Delay1/1
  [p_clt_1] -> Mux1/2
  Mux1/1 -> CL: (T2,p2,W2)/1
  Saturation1/1 -> Mux1/3, F0014_coreFlowDelay.m/1
  F0029_density.m/1 -> F0014_coreFlowDelay.m/2

== system component_lib/Thermal Systems/TH0005_flowSplit ==
  A (T1,p1,W1) : Inport
  split [-] : Inport  Port=2
  Demux1 : Demux  Outputs=3
  Mux1 : Mux  Inputs=3
  Mux2 : Mux  Inputs=3
  Product : Product
  Sum : Sum  Inputs=-+|
  B (T2,p2,W2) : Outport
  " C (T3,p3,W3)" : Outport  Port=2
  wires:
  Product/1 -> Mux1/3, Sum/1
  A (T1,p1,W1)/1 -> Demux1/1
  Demux1/3 -> Sum/2, Product/1
  Mux1/1 -> B (T2,p2,W2)/1
  split [-]/1 -> Product/2
  Mux2/1 -> " C (T3,p3,W3)"/1
  Sum/1 -> Mux2/3
  Demux1/1 -> [T_1]
  Demux1/2 -> Mux2/2, Mux1/2
  [T_1] -> Mux1/1
  [T_1] -> Mux2/1

== system component_lib/Thermal Systems/TH0006_flowConfluence ==
  note: Average pressure
  B (T1,p1,W1) : Inport
  C (T2,p2,W2) : Inport  Port=2
  Constant : Constant
  Demux1 : Demux  Outputs=3
  Demux2 : Demux  Outputs=3
  Gain : Gain  Gain=gain
  Gain1 : Gain  Gain=1/2
  Integrator Limited : Integrator  InitialCondition=0.5  LimitOutput=on  UpperSaturationLimit=1  LowerSaturationLimit=0
  Mux1 : Mux  Inputs=3
  Product : Product
  Product1 : Product
  Sum : Sum  Inputs=|+-
  Sum1 : Sum  Inputs=|++
  Sum2 : Sum  Inputs=++|
  Sum3 : Sum  Inputs=-+|
  Sum4 : Sum  Inputs=|++
  A (T3,p3,W3) : Outport
  split [-] : Outport  Port=2
  wires:
  B (T1,p1,W1)/1 -> Demux1/1
  Mux1/1 -> A (T3,p3,W3)/1
  C (T2,p2,W2)/1 -> Demux2/1
  Sum/1 -> Gain/1
  Gain/1 -> Integrator Limited/1
  Integrator Limited/1 -> split [-]/1, Product/2, Sum3/1
  Demux1/1 -> [T_11]
  Demux2/1 -> [T_12]
  Demux1/3 -> Sum1/1
  Sum1/1 -> Mux1/3
  Demux2/3 -> Sum1/2
  Demux1/2 -> [p_11]
  Demux2/2 -> [p_12]
  [p_11] -> Sum/1
  [p_12] -> Sum/2
  [T_11] -> Product/1
  Product/1 -> Sum2/1
  Product1/1 -> Sum2/2
  Sum2/1 -> Mux1/1
  Constant/1 -> Sum3/2
  [p_11] -> Sum4/1
  Sum4/1 -> Gain1/1
  [p_12] -> Sum4/2
  Gain1/1 -> Mux1/2
  Sum3/1 -> Product1/1
  [T_12] -> Product1/2

== system component_lib/Thermal Systems/TH0007_airRestriction ==
  AIR: (T1,p1,W1) : Inport
  Demux1 : Demux  Outputs=3
  F0014_restrictionPressureDrop2.m : base_lib/F0014_titanXradiator/F0014_restrictionPressureDrop2.m  SystemSampleTime=-1  VariantActivationTime=update diagram  Latency=0  AutoFrameSizeCalculation=off
      settings: LibrarySourceBlock=|
      | simulink/User-Defined
      | Functions/MATLAB Function
  Mux1 : Mux  Inputs=3
  Sum : Sum  Inputs=-+|
  AIR: (T2,p2,W2) : Outport
  wires:
  Mux1/1 -> AIR: (T2,p2,W2)/1
  AIR: (T1,p1,W1)/1 -> Demux1/1
  Demux1/3 -> F0014_restrictionPressureDrop2.m/3, Mux1/3
  Demux1/1 -> F0014_restrictionPressureDrop2.m/1, Mux1/1
  F0014_restrictionPressureDrop2.m/1 -> Sum/1
  Sum/1 -> Mux1/2
  Demux1/2 -> F0014_restrictionPressureDrop2.m/2, Sum/2

== system component_lib/Thermal Systems/TH0008_condenser ==
  AIR: (T1,p1,W1) : Inport
  Q [J/s] : Inport  Port=2
  AIrCp : Constant  Value=par.cp_air
  Demux1 : Demux  Outputs=3
  F0014_condenserPressureDrop.m : base_lib/F0014_titanXradiator/F0014_condenserPressureDrop.m  SystemSampleTime=-1  VariantActivationTime=update diagram  Latency=0  AutoFrameSizeCalculation=off
  Mux1 : Mux  Inputs=3
  Product3 : Product  Inputs=*//
  Saturation : Saturate  UpperLimit=inf  LowerLimit=0.001
  Saturation1 : Saturate  UpperLimit=373  LowerLimit=0
  Sum : Sum  Inputs=|+-
  Sum1 : Sum  Inputs=++|
  AIR: (T2,p2,W2) : Outport
  wires:
  AIR: (T1,p1,W1)/1 -> Demux1/1
  Mux1/1 -> AIR: (T2,p2,W2)/1
  Q [J/s]/1 -> Product3/1
  AIrCp/1 -> Product3/3
  Product3/1 -> Sum1/2  "dT"
  Demux1/1 -> [T_1]
  Saturation/1 -> Product3/2
  Demux1/3 -> Mux1/3, F0014_condenserPressureDrop.m/3, Saturation/1
  Sum1/1 -> Saturation1/1
  Saturation1/1 -> Mux1/1
  Demux1/2 -> [p_1]
  [p_1] -> F0014_condenserPressureDrop.m/2
  [T_1] -> F0014_condenserPressureDrop.m/1
  [p_1] -> Sum/1
  Sum/1 -> Mux1/2
  F0014_condenserPressureDrop.m/1 -> Sum/2
  [T_1] -> Sum1/1

== system component_lib/Thermal Systems/TH0009_intake ==
  AIR: (T1,p1,W1) : Inport
  v [m/s] : Inport  Port=2
  Demux1 : Demux  Outputs=3
  F0014_intakePressureIncrease.m : base_lib/F0014_titanXradiator/F0014_intakePressureIncrease.m  SystemSampleTime=-1  VariantActivationTime=update diagram  Latency=0  AutoFrameSizeCalculation=off
  Mux1 : Mux  Inputs=3
  Saturation : Saturate  UpperLimit=inf  LowerLimit=0
  Sum : Sum  Inputs=++|
  AIR: (T2,p2,W2) : Outport
  wires:
  Mux1/1 -> AIR: (T2,p2,W2)/1
  AIR: (T1,p1,W1)/1 -> Demux1/1
  Sum/1 -> Mux1/2
  Demux1/2 -> Sum/2, F0014_intakePressureIncrease.m/2
  F0014_intakePressureIncrease.m/1 -> Sum/1
  Demux1/3 -> Mux1/3
  Demux1/1 -> Mux1/1, F0014_intakePressureIncrease.m/1
  v [m/s]/1 -> Saturation/1
  Saturation/1 -> F0014_intakePressureIncrease.m/3

== system component_lib/Thermal Systems/TH0010_fan ==
  note: Density
  AIR: (T1,p1,W1) : Inport
  rel_speed [-] : Inport  Port=2
  Constant : Constant  Value=286
  Constant1 : Constant  Value=par.n_fan
  Constant2 : Constant  Value=par.dp0
  Constant3 : Constant  Value=3
  Constant4 : Constant  Value=par.P_nom
  Constant5 : Constant  Value=par.n_fan
  Demux1 : Demux  Outputs=3
  Divide : Product  Inputs=*//
  Divide1 : Product  Inputs=*//
  Divide2 : Product  Inputs=*/
  F0014_fanCurve.m : base_lib/F0014_titanXradiator/F0014_fanCurve.m  SystemSampleTime=-1  VariantActivationTime=update diagram  Latency=0  AutoFrameSizeCalculation=off
  Math Function : Math  Operator=square
  Math Function1 : Math  Operator=pow
  Mux : Mux  Inputs=3
  Product : Product
  Product1 : Product
  Product2 : Product  Inputs=3
  Ref. density : Constant  Value=1.18
  Sum : Sum  Inputs=|++
  Transfer Fcn : TransferFcn  Denominator=[0.1 1]
  AIR: (T2,p2,W2) : Outport
  P_fan [J/s] : Outport  Port=2
  wires:
  AIR: (T1,p1,W1)/1 -> Demux1/1
  Mux/1 -> AIR: (T2,p2,W2)/1
  Demux1/3 -> Mux/3, Divide/1
  Demux1/1 -> Mux/1, [T_1]
  [T_1] -> Divide1/2
  Constant/1 -> Divide1/3
  Divide1/1 -> Divide2/1, Divide/3
  Constant1/1 -> Divide/2
  Math Function/1 -> Product/1
  Constant2/1 -> Product/2
  Divide/1 -> F0014_fanCurve.m/1
  Product/1 -> F0014_fanCurve.m/2
  F0014_fanCurve.m/1 -> Product1/1
  Ref. density/1 -> Divide2/2
  Divide2/1 -> Product1/2
  Demux1/2 -> [p_1], Sum/1
  Product1/1 -> Sum/2
  Sum/1 -> Mux/2
  [p_1] -> Divide1/1
  Transfer Fcn/1 -> Math Function/1, Math Function1/1
  rel_speed [-]/1 -> Transfer Fcn/1
  Constant3/1 -> Math Function1/2
  Math Function1/1 -> Product2/1
  Constant4/1 -> Product2/2
  Product2/1 -> P_fan [J/s]/1
  Constant5/1 -> Product2/3

== system component_lib/Thermal Systems/TH0011_coolingChannel ==
  T_w [K] : Inport
  CL: (T1,p1,W1) : Inport  Port=2
  Demux : Demux  Outputs=3
  F0017_Nusselt.m : base_lib/F0017_channelCooling/F0017_Nusselt.m  SystemSampleTime=-1  VariantActivationTime=update diagram  Latency=0  AutoFrameSizeCalculation=off
  F0017_Prandtl.m : base_lib/F0017_channelCooling/F0017_Prandtl.m  SystemSampleTime=-1  VariantActivationTime=update diagram  Latency=0  AutoFrameSizeCalculation=off
  F0017_Reynolds.m : base_lib/F0017_channelCooling/F0017_Reynolds.m  SystemSampleTime=-1  VariantActivationTime=update diagram  Latency=0  AutoFrameSizeCalculation=off
  F0017_heatTransfer.m : base_lib/F0017_channelCooling/F0017_heatTransfer.m  SystemSampleTime=-1  VariantActivationTime=update diagram  Latency=0  AutoFrameSizeCalculation=off
  F0017_pressureDrop.m : base_lib/F0017_channelCooling/F0017_pressureDrop.m  SystemSampleTime=-1  VariantActivationTime=update diagram  Latency=0  AutoFrameSizeCalculation=off
  F0017_velocity.m : base_lib/F0017_channelCooling/F0017_velocity.m  SystemSampleTime=-1  VariantActivationTime=update diagram  Latency=0  AutoFrameSizeCalculation=off
  F0029_density.m : base_lib/F0029_coolantWrapper/F0029_density.m  SystemSampleTime=-1  VariantActivationTime=update diagram  Latency=0  AutoFrameSizeCalculation=off
      settings: LibrarySourceBlock=|
      | simulink/User-Defined
      | Functions/MATLAB Function
  F0029_heatCapacity.m : base_lib/F0029_coolantWrapper/F0029_heatCapacity.m  SystemSampleTime=-1  VariantActivationTime=update diagram  Latency=0  AutoFrameSizeCalculation=off
      settings: LibrarySourceBlock=|
      | simulink/User-Defined
      | Functions/MATLAB Function
  F0029_thermalConductivity.m : base_lib/F0029_coolantWrapper/F0029_thermalConductivity.m  SystemSampleTime=-1  VariantActivationTime=update diagram  Latency=0  AutoFrameSizeCalculation=off
      settings: LibrarySourceBlock=|
      | simulink/User-Defined
      | Functions/MATLAB Function
  F0029_viscosity.m : base_lib/F0029_coolantWrapper/F0029_viscosity.m  SystemSampleTime=-1  VariantActivationTime=update diagram  Latency=0  AutoFrameSizeCalculation=off
      settings: LibrarySourceBlock=|
      | simulink/User-Defined
      | Functions/MATLAB Function
  Gain : Gain  Gain=1/n_ch
  Gain1 : Gain  Gain=n_ch
  Gain2 : Gain  Gain=n_ch
  Mux : Mux  Inputs=3
  Sum : Sum  Inputs=-+|
  Q [J/s] : Outport
  CL: (T2,p2,W2) : Outport  Port=2
  wires:
  CL: (T1,p1,W1)/1 -> Demux/1
  Mux/1 -> CL: (T2,p2,W2)/1
  F0017_velocity.m/1 -> F0017_pressureDrop.m/1, F0017_Reynolds.m/1
  F0017_Reynolds.m/1 -> F0017_pressureDrop.m/2, F0017_Nusselt.m/1
  F0017_Prandtl.m/1 -> F0017_Nusselt.m/2
  Demux/1 -> F0029_density.m/1, F0029_viscosity.m/1, F0029_heatCapacity.m/1, F0029_thermalConductivity.m/1, F0017_heatTransfer.m/1
  T_w [K]/1 -> F0017_heatTransfer.m/2
  F0017_Nusselt.m/1 -> F0017_heatTransfer.m/3
  Sum/1 -> [p_2]
  [p_2] -> Mux/2
  Demux/2 -> Sum/2
  Demux/3 -> Gain/1
  F0017_pressureDrop.m/1 -> Sum/1
  F0017_heatTransfer.m/1 -> Gain2/1
  F0017_heatTransfer.m/2 -> Mux/1
  Gain/1 -> F0017_velocity.m/1, Gain1/1, F0017_heatTransfer.m/4
  Gain1/1 -> Mux/3
  Gain2/1 -> Q [J/s]/1
  F0029_density.m/1 -> [rho]
  [rho] -> F0017_velocity.m/2
  [rho] -> F0017_Reynolds.m/2
  F0029_thermalConductivity.m/1 -> [lam]
  [lam] -> F0017_Prandtl.m/3
  F0029_viscosity.m/1 -> [mu]
  [mu] -> F0017_Prandtl.m/2
  F0029_heatCapacity.m/1 -> [cp]
  [mu] -> F0017_Reynolds.m/3
  [cp] -> F0017_Prandtl.m/1
  [rho] -> F0017_pressureDrop.m/3
  [lam] -> F0017_heatTransfer.m/6
  [cp] -> F0017_heatTransfer.m/5

== system component_lib/Thermal Systems/TH0011_outletFlowBalance ==
  AIR: (T1,p1,W1) : Inport
  p_amb [Pa] : Inport  Port=2
  Demux : Demux  Outputs=3
  Gain : Gain  Gain=gain
  Integrator Limited : Integrator  LimitOutput=on  LowerSaturationLimit=0
  Sum : Sum  Inputs=|+-
  Terminator : Terminator
  Terminator1 : Terminator
  W_inlet [kg/s] : Outport
  wires:
  AIR: (T1,p1,W1)/1 -> Demux/1
  Demux/2 -> Sum/1
  p_amb [Pa]/1 -> Sum/2
  Sum/1 -> Gain/1
  Gain/1 -> Integrator Limited/1
  Integrator Limited/1 -> W_inlet [kg/s]/1
  Demux/1 -> Terminator/1
  Demux/3 -> Terminator1/1

== system component_lib/Thermal Systems/TH0011_pipe ==
  CL: (T1,p1,W1) : Inport
  Constant : Constant  Value=par.L
  Demux : Demux  Outputs=3
  Divide : Product  Inputs=*/
  F0017_Reynolds.m : base_lib/F0017_channelCooling/F0017_Reynolds.m  SystemSampleTime=-1  VariantActivationTime=update diagram  Latency=0  AutoFrameSizeCalculation=off
      settings: LibrarySourceBlock=|
      | simulink/User-Defined
      | Functions/MATLAB Function
  F0017_pressureDrop.m : base_lib/F0017_channelCooling/F0017_pressureDrop.m  SystemSampleTime=-1  VariantActivationTime=update diagram  Latency=0  AutoFrameSizeCalculation=off
      settings: LibrarySourceBlock=|
      | simulink/User-Defined
      | Functions/MATLAB Function
  F0017_velocity.m : base_lib/F0017_channelCooling/F0017_velocity.m  SystemSampleTime=-1  VariantActivationTime=update diagram  Latency=0  AutoFrameSizeCalculation=off
      settings: LibrarySourceBlock=|
      | simulink/User-Defined
      | Functions/MATLAB Function
  F0029_density.m : base_lib/F0029_coolantWrapper/F0029_density.m  SystemSampleTime=-1  VariantActivationTime=update diagram  Latency=0  AutoFrameSizeCalculation=off
      settings: LibrarySourceBlock=|
      | simulink/User-Defined
      | Functions/MATLAB Function
  F0029_viscosity.m : base_lib/F0029_coolantWrapper/F0029_viscosity.m  SystemSampleTime=-1  VariantActivationTime=update diagram  Latency=0  AutoFrameSizeCalculation=off
      settings: LibrarySourceBlock=|
      | simulink/User-Defined
      | Functions/MATLAB Function
  Mux : Mux  Inputs=3
  Saturation : Saturate  UpperLimit=10  LowerLimit=0
  Saturation1 : Saturate  UpperLimit=inf  LowerLimit=1e4
  Sum : Sum  Inputs=|+-
  Variable Transport Delay : VariableTransportDelay  VariableDelayType=Variable transport delay  MaximumDelay=10  InitialOutput=T_0
  CL: (T2,p2,W2) : Outport
  wires:
  CL: (T1,p1,W1)/1 -> Demux/1
  Constant/1 -> Divide/1
  F0017_velocity.m/1 -> Divide/2, F0017_Reynolds.m/1, F0017_pressureDrop.m/1
  Divide/1 -> Saturation/1
  Demux/1 -> F0029_viscosity.m/1, F0029_density.m/1, Variable Transport Delay/1
  F0017_Reynolds.m/1 -> F0017_pressureDrop.m/2
  F0017_pressureDrop.m/1 -> Sum/2
  Saturation/1 -> Variable Transport Delay/2
  Variable Transport Delay/1 -> Mux/1
  Sum/1 -> Saturation1/1
  Mux/1 -> CL: (T2,p2,W2)/1
  Demux/3 -> F0017_velocity.m/1, Mux/3
  Demux/2 -> Sum/1
  Saturation1/1 -> Mux/2
  F0029_density.m/1 -> F0017_pressureDrop.m/3, F0017_Reynolds.m/2, F0017_velocity.m/2
  F0029_viscosity.m/1 -> F0017_Reynolds.m/3

== system component_lib/Thermal Systems/TH0011_thermalMass ==
  dQ [J/s] : Inport
  Constant : Constant  Value=m
  Constant1 : Constant  Value=cp
  Integrator : Integrator  InitialCondition=T_0
  Product : Product  Inputs=*//
  T [K] : Outport
  wires:
  Integrator/1 -> T [K]/1
  Product/1 -> Integrator/1
  dQ [J/s]/1 -> Product/1
  Constant/1 -> Product/2
  Constant1/1 -> Product/3

== system component_lib/Thermal Systems/TH0012_equalSplitMerge ==
  note: merge/distribute flow
  CL: (T1,p1,W1) : Inport
  Demux : Demux  Outputs=3
  Gain : Gain  Gain=n
  Mux : Mux  Inputs=3
  CL: (T2,p2,W2) : Outport
  wires:
  CL: (T1,p1,W1)/1 -> Demux/1
  Demux/3 -> Gain/1
  Demux/1 -> Mux/1
  Gain/1 -> Mux/3
  Demux/2 -> Mux/2
  Mux/1 -> CL: (T2,p2,W2)/1

== system component_lib/Thermal Systems/TH0014_valve ==
  open [-] : Inport
  CL: (T1,p1,W1) : Inport  Port=2
  split [-] : Inport  Port=3
  Constant : Constant  Value=par.d
  Constant1 : Constant
  Constant2 : Constant
  Constant3 : Constant  Value=par.d
  Demux : Demux  Outputs=3
  F0017_incompressibleRestriction.m : base_lib/F0017_channelCooling/F0017_incompressibleRestriction.m  SystemSampleTime=-1  VariantActivationTime=update diagram  Latency=0  AutoFrameSizeCalculation=off
      settings: LibrarySourceBlock=|
      | simulink/User-Defined
      | Functions/MATLAB Function
  F0017_incompressibleRestriction.m1 : base_lib/F0017_channelCooling/F0017_incompressibleRestriction.m  SystemSampleTime=-1  VariantActivationTime=update diagram  Latency=0  AutoFrameSizeCalculation=off
      settings: LibrarySourceBlock=|
      | simulink/User-Defined
      | Functions/MATLAB Function
  F0029_density.m : base_lib/F0029_coolantWrapper/F0029_density.m  SystemSampleTime=-1  VariantActivationTime=update diagram  Latency=0  AutoFrameSizeCalculation=off
      settings: LibrarySourceBlock=|
      | simulink/User-Defined
      | Functions/MATLAB Function
  Mux : Mux  Inputs=3
  Mux1 : Mux  Inputs=3
  Product{,1..3} (4 alike) : Product
  Saturation : Saturate  UpperLimit=1  LowerLimit=0
  Saturation1 : Saturate  UpperLimit=0.99  LowerLimit=0.01
  Sum : Sum  Inputs=-+|
  Sum1 : Sum  Inputs=-+|
  Sum2 : Sum  Inputs=|+-
  Sum3 : Sum  Inputs=|+-
  Transfer Fcn : TransferFcn  Denominator=[0.1 1]
  CL: (T2,p2,W2) : Outport
  CL: (T3,p3,W3) : Outport  Port=2
  wires:
  CL: (T1,p1,W1)/1 -> Demux/1
  Mux/1 -> CL: (T2,p2,W2)/1
  Saturation1/1 -> Sum/1, Product/1
  Constant1/1 -> Sum/2
  Sum/1 -> Product1/2
  Constant2/1 -> Sum1/2
  Product2/1 -> F0017_incompressibleRestriction.m/1, [W_21]
  Product3/1 -> F0017_incompressibleRestriction.m1/1, [W_20]
  Sum1/1 -> Product3/2
  Demux/3 -> Product3/1, Product2/1
  Mux1/1 -> CL: (T3,p3,W3)/1
  Sum2/1 -> Mux/2
  F0017_incompressibleRestriction.m/1 -> Sum2/2
  Demux/1 -> F0029_density.m/1, Mux1/1, Mux/1
  [W_20] -> Mux1/3
  Demux/2 -> [p_1]
  Sum3/1 -> Mux1/2
  [p_1] -> Sum3/1
  F0017_incompressibleRestriction.m1/1 -> Sum3/2
  [p_1] -> Sum2/1
  [W_21] -> Mux/3
  Saturation/1 -> Sum1/1, Product2/2
  split [-]/1 -> Saturation/1
  open [-]/1 -> Transfer Fcn/1
  Transfer Fcn/1 -> Saturation1/1
  Constant/1 -> Product/2
  Constant3/1 -> Product1/1
  Product/1 -> F0017_incompressibleRestriction.m/2
  Product1/1 -> F0017_incompressibleRestriction.m1/2
  F0029_density.m/1 -> [rho]
  [rho] -> F0017_incompressibleRestriction.m/3
  [rho] -> F0017_incompressibleRestriction.m1/3

== system component_lib/Thermal Systems/TH0015_totalHeatTransfer ==
  Q [J/s] : Inport
  CL: (T1,p1,W1) : Inport  Port=2
  Demux : Demux  Outputs=3
  F0029_heatCapacity.m : base_lib/F0029_coolantWrapper/F0029_heatCapacity.m  SystemSampleTime=-1  VariantActivationTime=update diagram  Latency=0  AutoFrameSizeCalculation=off
      settings: LibrarySourceBlock=|
      | simulink/User-Defined
      | Functions/MATLAB Function
  Mux : Mux  Inputs=3
  Product : Product  Inputs=*//
  Saturation : Saturate  UpperLimit=T_max  LowerLimit=T_min
  Saturation1 : Saturate  UpperLimit=inf  LowerLimit=0.001
  Sum : Sum  Inputs=++|
  CL: (T2,p2,W2) : Outport
  wires:
  CL: (T1,p1,W1)/1 -> Demux/1
  Mux/1 -> CL: (T2,p2,W2)/1
  Demux/2 -> Mux/2
  Q [J/s]/1 -> Product/1
  F0029_heatCapacity.m/1 -> Product/3
  Demux/1 -> F0029_heatCapacity.m/1, Sum/2
  Product/1 -> Sum/1
  Sum/1 -> Saturation/1
  Saturation/1 -> Mux/1
  Demux/3 -> Saturation1/1, Mux/3
  Saturation1/1 -> Product/2

== system component_lib/Thermal Systems/TH0016_calculateHeatflow ==
  "CL: (T1, p1, W1)" : Inport
  "CL: (T2, p2, W2)" : Inport  Port=2
  Demux : Demux  Outputs=3
  Demux1 : Demux  Outputs=3
  F0029_heatCapacity.m : base_lib/F0029_coolantWrapper/F0029_heatCapacity.m  SystemSampleTime=-1  VariantActivationTime=update diagram  Latency=0  AutoFrameSizeCalculation=off
      settings: LibrarySourceBlock=|
      | simulink/User-Defined
      | Functions/MATLAB Function
  F0029_heatCapacity.m1 : base_lib/F0029_coolantWrapper/F0029_heatCapacity.m  SystemSampleTime=-1  VariantActivationTime=update diagram  Latency=0  AutoFrameSizeCalculation=off
      settings: LibrarySourceBlock=|
      | simulink/User-Defined
      | Functions/MATLAB Function
  Gain : Gain  Gain=1/2
  Product : Product  Inputs=3
  Sum : Sum  Inputs=|-+
  Sum1 : Sum  Inputs=|++
  Terminator : Terminator
  Terminator1 : Terminator
  Terminator2 : Terminator
  Q [J/s] : Outport
  wires:
  "CL: (T1, p1, W1)"/1 -> Demux/1
  "CL: (T2, p2, W2)"/1 -> Demux1/1
  Product/1 -> Q [J/s]/1
  Demux/2 -> Terminator/1
  Demux1/2 -> Terminator1/1
  Demux1/3 -> Terminator2/1
  Demux1/1 -> F0029_heatCapacity.m1/1, Sum/2
  Sum/1 -> Product/1
  Demux/1 -> F0029_heatCapacity.m/1, Sum/1
  Demux/3 -> Product/3
  F0029_heatCapacity.m/1 -> Sum1/1
  F0029_heatCapacity.m1/1 -> Sum1/2
  Sum1/1 -> Gain/1
  Gain/1 -> Product/2

== system component_lib/Thermal Systems/TH0017_calculateHeatflow ==
  "AIR: (T1, p1, W1)" : Inport
  "AIR: (T2, p2, W2)" : Inport  Port=2
  Constant2 : Constant  Value=par.cp_air
  Demux : Demux  Outputs=3
  Demux1 : Demux  Outputs=3
  Product : Product  Inputs=3
  Sum : Sum  Inputs=|-+
  Terminator : Terminator
  Terminator1 : Terminator
  Terminator2 : Terminator
  Q [J/s] : Outport
  wires:
  "AIR: (T1, p1, W1)"/1 -> Demux/1
  "AIR: (T2, p2, W2)"/1 -> Demux1/1
  Constant2/1 -> Product/2
  Product/1 -> Q [J/s]/1
  Demux/2 -> Terminator/1
  Demux1/2 -> Terminator1/1
  Demux1/3 -> Terminator2/1
  Demux1/1 -> Sum/2
  Sum/1 -> Product/1
  Demux/1 -> Sum/1
  Demux/3 -> Product/3
